simulink model "sim_model_simpledclink_2parallel_rlload"  (R2016a)
settings: Solver=ode4  StartTime=0.0  StopTime=Tfinal  FixedStep=Ts  RelTol=1e-3
values from neighbouring files (symbols this model uses):
  Cdc = 3*Cdc1    (= 1.5e-05)    [sim_parameters.m]    (also in sim_parameters_parallel.m; sim_parameters_rl_load.m)
  delta = acos(Ef/Vt)    [sim_parameters.m]    (also in sim_parameters_parallel.m; sim_parameters_rl_load.m = 0)
  deltad = delta*180/pi    [sim_parameters.m]    (also in sim_parameters_parallel.m; sim_parameters_rl_load.m = 0)
  ESL = 19e-9    (= 1.9e-08)    [sim_parameters.m]    (also in sim_parameters_parallel.m = 1.9e-14; sim_parameters_rl_load.m = 1e-15)
  ESR = 21.1e-15    (= 2.11e-14)    [sim_parameters_parallel.m]    (also in sim_parameters_rl_load.m = 1e-15)
  Lin = 1e-15    [sim_parameters_parallel.m]    (also in sim_parameters_rl_load.m = 1e-06)
  Lload = Xload/(2*pi*fout)    [sim_parameters_rl_load.m]
  ma = Vt*sqrt(3)/(Vdcm*0.612)    [sim_parameters.m]    (also in sim_parameters_parallel.m; sim_parameters_rl_load.m = 0.9)
  maxlim = 340    [sim_parameters.m]    (also in sim_parameters_parallel.m; sim_parameters_rl_load.m)
  minlim = 200    [sim_parameters.m]    (also in sim_parameters_parallel.m; sim_parameters_rl_load.m)
  phase = [0 90 0 90]    [sim_parameters.m]    (also in sim_parameters_parallel.m = [0 0]; sim_parameters_rl_load.m = [0 0])
  Rin = 1    [sim_parameters.m]    (also in sim_parameters_parallel.m = 50; sim_parameters_rl_load.m = 200)
  Ripth = 0.25    [sim_parameters.m]    (also in sim_parameters_parallel.m = 0.3; sim_parameters_rl_load.m = 0.03)
  Rload = Zload*pf    [sim_parameters_rl_load.m]
  Ts = 1e-6    (= 1e-06)    [sim_parameters.m]    (also in sim_parameters_parallel.m = 1e-07; sim_parameters_rl_load.m = 1e-08)
  Vin = Vdc + Rin*(Pout/Vdc)    (= 1751.48148148)    [sim_parameters_rl_load.m]
  wout = 2*pi*fout    (= 314.159265359)    [sim_parameters.m]    (also in sim_parameters_parallel.m; sim_parameters_rl_load.m)
libraries: powerlib x39, powerlib_meascontrol x26, simulink x2
settings Model: SimulationMode=accelerator  Creator=ugurm  LastModifiedBy=mesutto
settings DataIOCC: LimitDataPoints=on  SaveFormat=Array
settings DebuggingCC: UnderspecifiedInitializationDetection=Classic  MergeDetectMultiDrivingBlocksExec=none  SolverPrmCheckMsg=warning  StateNameClashWarn=warning
settings HardwareCC: ProdBitPerPointer=32  ProdLargestAtomicFloat=None  ProdIntDivRoundTo=Undefined  ProdEndianess=Unspecified  ProdWordSize=32  ProdHWDeviceType=32-bit Generic
settings ModelReferenceCC: PropagateSignalLabelsOutOfModel=off
settings ConfigComp: CovModelRefEnable=Off

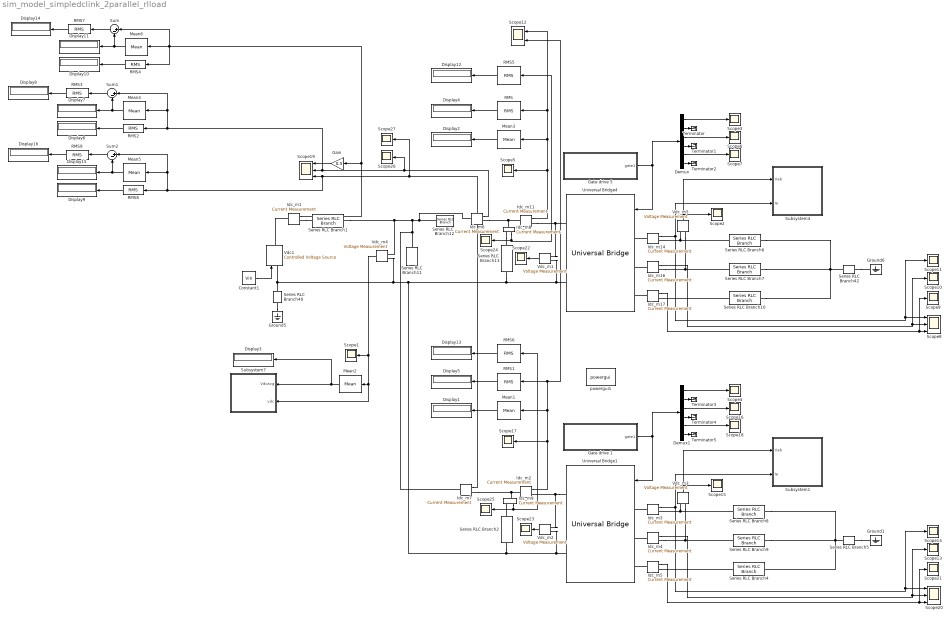
== system sim_model_simpledclink_2parallel_rlload ==
  Constant1 : Constant  Value=Vin
  Demux : Demux  Outputs=6
  Demux1 : Demux  Outputs=6
  Display{1..16} (16 alike) : Display
  Gain : Gain  Gain=0.5
  Gate drive 1 : Subsystem
  Gate drive 5 : Subsystem
  Ground1 : powerlib/Elements/Ground  LConnTagsString=a
  Ground5 : powerlib/Elements/Ground  LConnTagsString=a
  Ground6 : powerlib/Elements/Ground  LConnTagsString=a
  Idc_m{1..9,11,14,16..17} (13 alike) : powerlib/Measurements/Current Measurement  PhasorSimulation=off  OutputType=Complex  PSBequivalent=0
  Mean{1..6} (6 alike) : powerlib_meascontrol/Measurements/Mean  Freq=fout  Vinit=0  Ts=0
  RMS{,1..9} (10 alike) : powerlib_meascontrol/Measurements/RMS  TrueRMS=on  Freq=fout  RMSInit=0  Ts=0
  Scope{1..7,9..11,13..18,21..27} (23 alike) : Scope
  Scope12 : Scope  NumInputPorts=2
  Scope19 : Scope  NumInputPorts=3
  Scope20 : Scope  NumInputPorts=3
  Scope8 : Scope  NumInputPorts=3
  Series RLC Branch1 : powerlib/Elements/Series RLC Branch  LConnTagsString=__new0  RConnTagsString=__new0  BranchType=R  Resistance=Rin  Inductance=Lin  SetiL0=off  InitialCurrent=0  Capacitance=1e-6  Setx0=off  InitialVoltage=0  Measurements=None
  Series RLC Branch{4,6..10} (6 alike) : powerlib/Elements/Series RLC Branch  LConnTagsString=__new0  RConnTagsString=__new0  BranchType=RL  Resistance=Rload  Inductance=Lload  SetiL0=off  InitialCurrent=0  Capacitance=1e-6  Setx0=off  InitialVoltage=0  Measurements=None
  Series RLC Branch11 : powerlib/Elements/Series RLC Branch  LConnTagsString=__new0  RConnTagsString=__new0  BranchType=RL  Resistance=1e-3  Inductance=1e-6  SetiL0=off  InitialCurrent=0  Capacitance=1e-6  Setx0=off  InitialVoltage=0  Measurements=None
  Series RLC Branch12 : powerlib/Elements/Series RLC Branch  LConnTagsString=__new0  RConnTagsString=__new0  BranchType=RL  Resistance=1e-3  Inductance=1e-6  SetiL0=off  InitialCurrent=0  Capacitance=1e-6  Setx0=off  InitialVoltage=0  Measurements=None
  Series RLC Branch13 : powerlib/Elements/Series RLC Branch  LConnTagsString=__new0  RConnTagsString=__new0  BranchType=RLC  Resistance=ESR  Inductance=ESL  SetiL0=off  InitialCurrent=0  Capacitance=Cdc  Setx0=off  InitialVoltage=0  Measurements=None
  Series RLC Branch2 : powerlib/Elements/Series RLC Branch  LConnTagsString=__new0  RConnTagsString=__new0  BranchType=RLC  Resistance=ESR  Inductance=ESL  SetiL0=off  InitialCurrent=0  Capacitance=Cdc  Setx0=off  InitialVoltage=0  Measurements=None
  Series RLC Branch40 : powerlib/Elements/Series RLC Branch  LConnTagsString=__new0  RConnTagsString=__new0  BranchType=R  Resistance=1e12  Inductance=Lload  SetiL0=off  InitialCurrent=0  Capacitance=1e-6  Setx0=off  InitialVoltage=0  Measurements=None
  Series RLC Branch42 : powerlib/Elements/Series RLC Branch  LConnTagsString=__new0  RConnTagsString=__new0  BranchType=R  Resistance=1e12  Inductance=Lload  SetiL0=off  InitialCurrent=0  Capacitance=1e-6  Setx0=off  InitialVoltage=0  Measurements=None
  Series RLC Branch5 : powerlib/Elements/Series RLC Branch  LConnTagsString=__new0  RConnTagsString=__new0  BranchType=R  Resistance=1e12  Inductance=Lload  SetiL0=off  InitialCurrent=0  Capacitance=1e-6  Setx0=off  InitialVoltage=0  Measurements=None
  Subsystem1 : Subsystem
  Subsystem4 : Subsystem
  Subsystem7 : Subsystem
  Sum : Sum  Inputs=|+-
  Sum1 : Sum  Inputs=|+-
  Sum2 : Sum  Inputs=|+-
  Terminator{,1..5} (6 alike) : Terminator
  Universal Bridge1 : powerlib/Power Electronics/Universal Bridge  Arms=3  SnubberResistance=1e5  SnubberCapacitance=inf  Device=IGBT / Diodes  Ron=1e-6  Lon=0  ForwardVoltages="[  0  0  ]"  ForwardVoltage=0  GTOparameters=[ 10e-6 , 20e-6 ]  IGBTparameters=[0,0]  Measurements=None  Measurements_2=None  converterType=Rectifier
  Universal Bridge4 : powerlib/Power Electronics/Universal Bridge  Arms=3  SnubberResistance=1e5  SnubberCapacitance=inf  Device=IGBT / Diodes  Ron=1e-6  Lon=0  ForwardVoltages="[  0  0  ]"  ForwardVoltage=0  GTOparameters=[ 10e-6 , 20e-6 ]  IGBTparameters=[0,0]  Measurements=None  Measurements_2=None  converterType=Rectifier
  Vdc1 : powerlib/Electrical Sources/Controlled Voltage Source  Initialize=off  Source_Type=DC  Amplitude=200  Phase=0  Frequency=0  Measurements=None
  Vdc_m{1..5} (5 alike) : powerlib/Measurements/Voltage Measurement  PhasorSimulation=off  OutputType=Complex  PSBequivalent=0
  powergui1 : powerlib/powergui  Priority=1  SimulationMode=Discrete  SolverType=Tustin  SampleTime=Ts  frequency=60  SPID=off  DisableSnubberDevices=off  DisableRonSwitches=off  DisableVfSwitches=off  SwTol=0  DisplayEquations=off  Interpol=off  ExternalGateDelay=off  methode=off  Ts=0  FunctionMessages=off  echomessages=off  HookPort=off  EnableUseOfTLC=off  x0status=blocks  frequencyindice=0  Pbase=100e6  ErrMax=1e-4  Iterations=50  UnitsV=kV  UnitsW=MW  buscounter=0  RestoreLinks=warning  ResistiveCurrentMeasurement=off  Frange=[0:2:500]  Ylog=off  Xlog=on  ShowGrid=off  save=off  variable=ZData  structure=vdc  ZoomFFT=off  StartTime=0.35  cycles=5  DisplayStyle=4  fundamental=50  FreqAxis=off  MaxFrequency=50000  frequencyindicesteady=1  RmsSteady=1  display=off
  wires:
  Gate drive 5/1(gate1) -> Universal Bridge4/1, Demux/1
  Vdc_m5/1 -> Subsystem4/1(Vab), Scope2/1
  Idc_m14/1 -> Subsystem4/2(Ia), Scope11/1, Scope8/1
  Constant1/1 -> Vdc1/1
  Idc_m16/1 -> Scope10/1, Scope8/2
  Idc_m17/1 -> Scope9/1, Scope8/3
  Idc_m11/1 -> Mean3/1, RMS/1, Scope12/1, Scope5/1
  Mean3/1 -> Display2/1
  RMS/1 -> Display4/1
  Demux/1 -> Scope3/1
  Demux/5 -> Scope7/1
  Demux/3 -> Scope6/1
  Demux/2 -> Terminator/1
  Demux/4 -> Terminator1/1
  Demux/6 -> Terminator2/1
  Mean2/1 -> Display3/1, Subsystem7/1(Vdcavg)
  Gate drive 1/1(gate1) -> Universal Bridge1/1, Demux1/1
  Vdc_m3/1 -> Subsystem1/1(Vab), Scope15/1
  Idc_m3/1 -> Subsystem1/2(Ia), Scope14/1, Scope20/1
  Idc_m4/1 -> Scope13/1, Scope20/2
  Idc_m5/1 -> Scope21/1, Scope20/3
  Idc_m2/1 -> Mean1/1, Scope12/2, RMS1/1, Scope17/1
  Mean1/1 -> Display1/1
  RMS1/1 -> Display5/1
  Demux1/1 -> Scope4/1
  Demux1/5 -> Scope18/1
  Demux1/3 -> Scope16/1
  Demux1/2 -> Terminator3/1
  Demux1/4 -> Terminator4/1
  Demux1/6 -> Terminator5/1
  Vdc_m4/1 -> Scope1/1, Subsystem7/2(vdc), Mean2/1
  Gain/1 -> Scope19/1
  Vdc_m1/1 -> Scope22/1
  Vdc_m2/1 -> Scope23/1
  Idc_m8/1 -> RMS5/1, Scope24/1
  Idc_m6/1 -> Sum1/1, Mean4/1, RMS2/1, Scope19/2, Scope26/1
  RMS4/1 -> Display10/1
  Idc_m1/1 -> Sum/1, RMS4/1, Mean6/1, Gain/1
  Mean6/1 -> Display11/1, Sum/2
  RMS5/1 -> Display12/1
  RMS6/1 -> Display13/1
  Idc_m9/1 -> RMS6/1, Scope25/1
  Sum/1 -> RMS7/1
  RMS7/1 -> Display14/1
  RMS2/1 -> Display6/1
  Mean4/1 -> Display7/1, Sum1/2
  Sum1/1 -> RMS3/1
  RMS3/1 -> Display8/1
  RMS8/1 -> Display9/1
  Idc_m7/1 -> Scope27/1, Mean5/1, Sum2/1, RMS8/1, Scope19/3
  Mean5/1 -> Display15/1, Sum2/2
  Sum2/1 -> RMS9/1
  RMS9/1 -> Display16/1
  connections:
  Vdc_m5/LConn1 -- Series RLC Branch6/LConn1 -- Idc_m14/RConn1
  Series RLC Branch42/RConn1 -- Ground6/LConn1
  Series RLC Branch40/RConn1 -- Ground5/LConn1
  Idc_m14/LConn1 -- Universal Bridge4/LConn1
  Series RLC Branch42/LConn1 -- Series RLC Branch7/RConn1 -- Series RLC Branch10/RConn1 -- Series RLC Branch6/RConn1
  Idc_m16/LConn1 -- Universal Bridge4/LConn2
  Idc_m17/LConn1 -- Universal Bridge4/LConn3
  Series RLC Branch10/LConn1 -- Idc_m17/RConn1
  Idc_m16/RConn1 -- Series RLC Branch7/LConn1 -- Vdc_m5/LConn2
  Idc_m11/RConn1 -- Vdc_m1/LConn1 -- Universal Bridge4/RConn1
  Idc_m1/RConn1 -- Series RLC Branch1/LConn1
  Idc_m1/LConn1 -- Vdc1/RConn1
  Idc_m3/RConn1 -- Series RLC Branch8/LConn1 -- Vdc_m3/LConn1
  Vdc_m3/LConn2 -- Series RLC Branch9/LConn1 -- Idc_m4/RConn1
  Universal Bridge4/RConn2 -- Vdc_m1/LConn2 -- Series RLC Branch13/RConn1 -- Series RLC Branch2/RConn1 -- Universal Bridge1/RConn2 -- Vdc_m2/LConn2 -- Vdc_m4/LConn2 -- Vdc1/LConn1 -- Series RLC Branch40/LConn1
  Universal Bridge1/RConn1 -- Idc_m2/RConn1 -- Vdc_m2/LConn1
  Idc_m7/RConn1 -- Idc_m9/LConn1 -- Idc_m2/LConn1
  Idc_m3/LConn1 -- Universal Bridge1/LConn1
  Idc_m4/LConn1 -- Universal Bridge1/LConn2
  Series RLC Branch4/LConn1 -- Idc_m5/RConn1
  Idc_m5/LConn1 -- Universal Bridge1/LConn3
  Series RLC Branch5/RConn1 -- Ground1/LConn1
  Idc_m6/RConn1 -- Idc_m8/LConn1 -- Idc_m11/LConn1
  Vdc_m4/LConn1 -- Series RLC Branch1/RConn1 -- Idc_m6/LConn1 -- Series RLC Branch12/LConn1 -- Idc_m7/LConn1 -- Series RLC Branch11/RConn1
  Series RLC Branch8/RConn1 -- Series RLC Branch9/RConn1 -- Series RLC Branch5/LConn1 -- Series RLC Branch4/RConn1
  Idc_m8/RConn1 -- Series RLC Branch13/LConn1
  Series RLC Branch2/LConn1 -- Idc_m9/RConn1

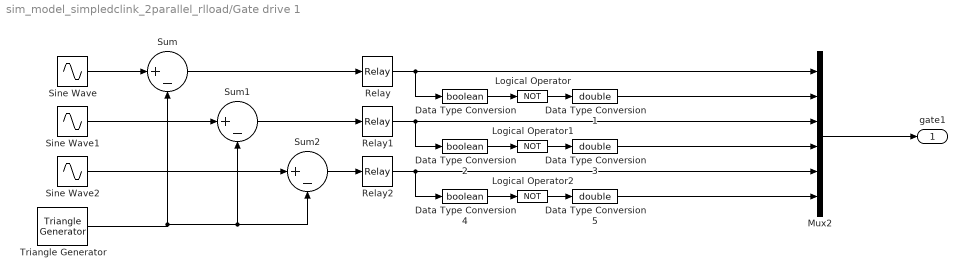
== system sim_model_simpledclink_2parallel_rlload/Gate drive 1 ==
  Data Type Conversion : DataTypeConversion  OutDataTypeStr=boolean
  Data Type Conversion1 : DataTypeConversion  OutDataTypeStr=double
  Data Type Conversion2 : DataTypeConversion  OutDataTypeStr=boolean
  Data Type Conversion3 : DataTypeConversion  OutDataTypeStr=double
  Data Type Conversion4 : DataTypeConversion  OutDataTypeStr=boolean
  Data Type Conversion5 : DataTypeConversion  OutDataTypeStr=double
  Logical Operator : Logic  Operator=NOT  AllPortsSameDT=off  OutDataTypeStr=boolean
  Logical Operator1 : Logic  Operator=NOT  AllPortsSameDT=off  OutDataTypeStr=boolean
  Logical Operator2 : Logic  Operator=NOT  AllPortsSameDT=off  OutDataTypeStr=boolean
  Mux2 : Mux  Inputs=6
  Relay : Relay
  Relay1 : Relay
  Relay2 : Relay
  Sine Wave : Sin  Amplitude=ma  Frequency=wout  Phase=delta  SampleTime=0
  Sine Wave1 : Sin  Amplitude=ma  Frequency=wout  Phase=-2*pi/3+delta  SampleTime=0
  Sine Wave2 : Sin  Amplitude=ma  Frequency=wout  Phase=2*pi/3+delta  SampleTime=0
  Sum : Sum  Inputs=|+-
  Sum1 : Sum  Inputs=|+-
  Sum2 : Sum  Inputs=|+-
  Triangle Generator : powerlib_meascontrol/Pulse & Signal Generators/Triangle Generator  Freq=fsw  Phase=phase(2)  Ts=Ts
  gate1 : Outport
  wires:
  Sine Wave/1 -> Sum/1
  Triangle Generator/1 -> Sum1/2, Sum2/2, Sum/2
  Sine Wave1/1 -> Sum1/1
  Sine Wave2/1 -> Sum2/1
  Sum/1 -> Relay/1
  Sum1/1 -> Relay1/1
  Sum2/1 -> Relay2/1
  Data Type Conversion/1 -> Logical Operator/1
  Relay/1 -> Data Type Conversion/1, Mux2/1
  Logical Operator/1 -> Data Type Conversion1/1
  Data Type Conversion1/1 -> Mux2/2
  Data Type Conversion2/1 -> Logical Operator1/1
  Relay1/1 -> Data Type Conversion2/1, Mux2/3
  Logical Operator1/1 -> Data Type Conversion3/1
  Data Type Conversion3/1 -> Mux2/4
  Data Type Conversion4/1 -> Logical Operator2/1
  Relay2/1 -> Data Type Conversion4/1, Mux2/5
  Logical Operator2/1 -> Data Type Conversion5/1
  Data Type Conversion5/1 -> Mux2/6
  Mux2/1 -> gate1/1

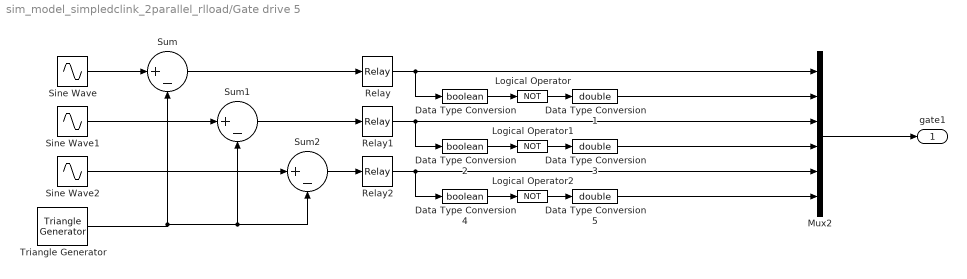
== system sim_model_simpledclink_2parallel_rlload/Gate drive 5 ==
  Data Type Conversion : DataTypeConversion  OutDataTypeStr=boolean
  Data Type Conversion1 : DataTypeConversion  OutDataTypeStr=double
  Data Type Conversion2 : DataTypeConversion  OutDataTypeStr=boolean
  Data Type Conversion3 : DataTypeConversion  OutDataTypeStr=double
  Data Type Conversion4 : DataTypeConversion  OutDataTypeStr=boolean
  Data Type Conversion5 : DataTypeConversion  OutDataTypeStr=double
  Logical Operator : Logic  Operator=NOT  AllPortsSameDT=off  OutDataTypeStr=boolean
  Logical Operator1 : Logic  Operator=NOT  AllPortsSameDT=off  OutDataTypeStr=boolean
  Logical Operator2 : Logic  Operator=NOT  AllPortsSameDT=off  OutDataTypeStr=boolean
  Mux2 : Mux  Inputs=6
  Relay : Relay
  Relay1 : Relay
  Relay2 : Relay
  Sine Wave : Sin  Amplitude=ma  Frequency=wout  Phase=delta  SampleTime=0
  Sine Wave1 : Sin  Amplitude=ma  Frequency=wout  Phase=-2*pi/3+delta  SampleTime=0
  Sine Wave2 : Sin  Amplitude=ma  Frequency=wout  Phase=2*pi/3+delta  SampleTime=0
  Sum : Sum  Inputs=|+-
  Sum1 : Sum  Inputs=|+-
  Sum2 : Sum  Inputs=|+-
  Triangle Generator : powerlib_meascontrol/Pulse & Signal Generators/Triangle Generator  Freq=fsw  Phase=phase(1)  Ts=Ts
  gate1 : Outport
  wires:
  Sine Wave/1 -> Sum/1
  Triangle Generator/1 -> Sum1/2, Sum2/2, Sum/2
  Sine Wave1/1 -> Sum1/1
  Sine Wave2/1 -> Sum2/1
  Sum/1 -> Relay/1
  Sum1/1 -> Relay1/1
  Sum2/1 -> Relay2/1
  Data Type Conversion/1 -> Logical Operator/1
  Relay/1 -> Data Type Conversion/1, Mux2/1
  Logical Operator/1 -> Data Type Conversion1/1
  Data Type Conversion1/1 -> Mux2/2
  Data Type Conversion2/1 -> Logical Operator1/1
  Relay1/1 -> Data Type Conversion2/1, Mux2/3
  Logical Operator1/1 -> Data Type Conversion3/1
  Data Type Conversion3/1 -> Mux2/4
  Data Type Conversion4/1 -> Logical Operator2/1
  Relay2/1 -> Data Type Conversion4/1, Mux2/5
  Logical Operator2/1 -> Data Type Conversion5/1
  Data Type Conversion5/1 -> Mux2/6
  Mux2/1 -> gate1/1

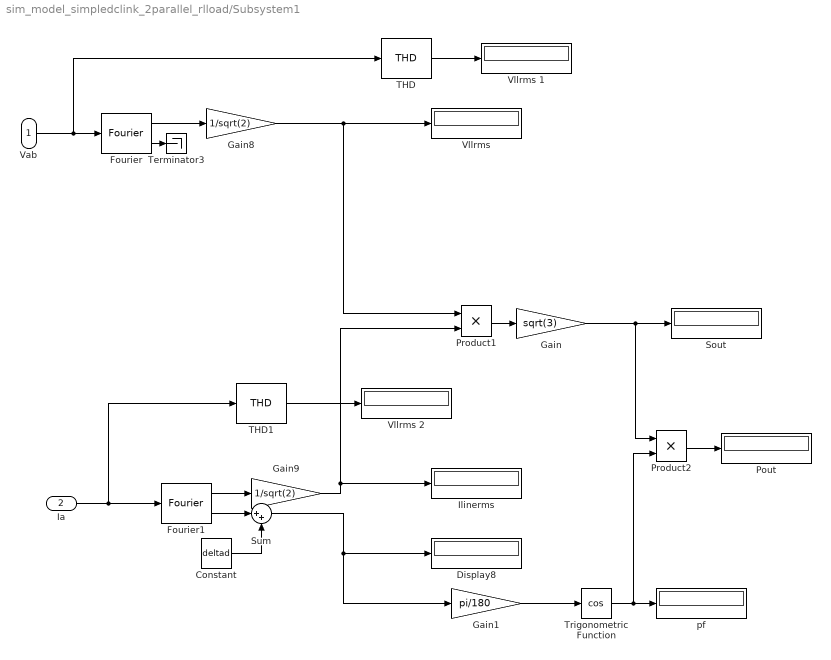
== system sim_model_simpledclink_2parallel_rlload/Subsystem1 ==
  Vab : Inport
  Ia : Inport  Port=2
  Constant : Constant  Value=deltad
  Display8 : Display
  Fourier : powerlib_meascontrol/Measurements/Fourier  Freq=fout  n=1  InInit=[0, 0]  Ts=Ts
  Fourier1 : powerlib_meascontrol/Measurements/Fourier  Freq=fout  n=1  InInit=[0, 0]  Ts=Ts
  Gain : Gain  Gain=sqrt(3)
  Gain1 : Gain  Gain=pi/180
  Gain8 : Gain  Gain=1/sqrt(2)
  Gain9 : Gain  Gain=1/sqrt(2)
  "Ilinerms " : Display
  Pout : Display
  Product1 : Product
  Product2 : Product
  Sout : Display
      settings: Format=short_e
  Sum : Sum  Inputs=|++
  THD : powerlib_meascontrol/Measurements/THD  Freq=fout  Ts=0
  THD1 : powerlib_meascontrol/Measurements/THD  Freq=fout  Ts=0
  Terminator3 : Terminator
  Trigonometric Function : Trigonometry  Operator=cos
  "Vllrms " : Display
  Vllrms 1 : Display
  Vllrms 2 : Display
  pf : Display
  wires:
  Gain8/1 -> Product1/1, "Vllrms "/1
  Gain9/1 -> "Ilinerms "/1, Product1/2
  Ia/1 -> THD1/1, Fourier1/1
  Fourier1/1 -> Gain9/1
  Vab/1 -> THD/1, Fourier/1
  Fourier/1 -> Gain8/1
  Product1/1 -> Gain/1
  Gain/1 -> Product2/1, Sout/1
  Sum/1 -> Gain1/1, Display8/1
  Trigonometric Function/1 -> Product2/2, pf/1
  Gain1/1 -> Trigonometric Function/1
  Product2/1 -> Pout/1
  Fourier/2 -> Terminator3/1
  THD/1 -> Vllrms 1/1
  THD1/1 -> Vllrms 2/1
  Fourier1/2 -> Sum/1
  Constant/1 -> Sum/2

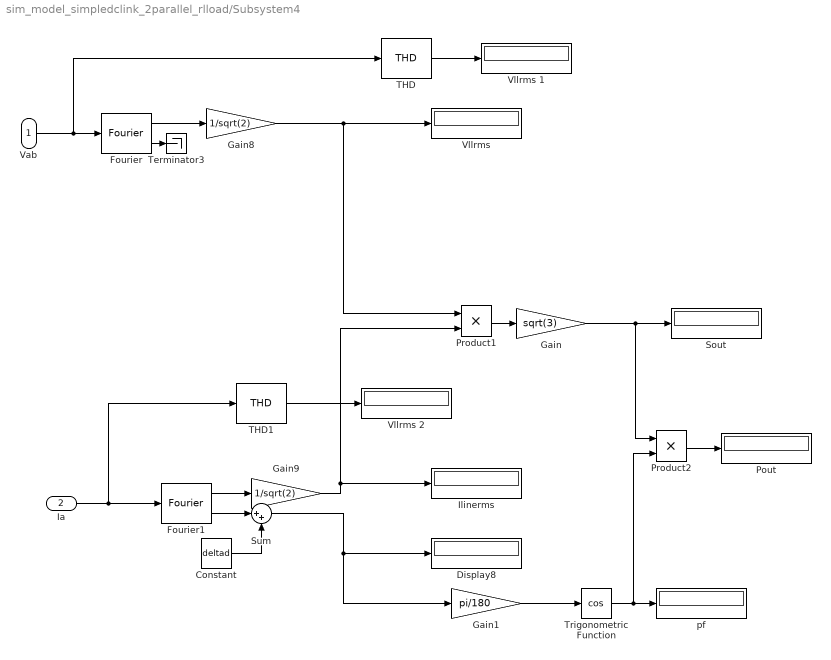
== system sim_model_simpledclink_2parallel_rlload/Subsystem4 ==
  Vab : Inport
  Ia : Inport  Port=2
  Constant : Constant  Value=deltad
  Display8 : Display
  Fourier : powerlib_meascontrol/Measurements/Fourier  Freq=fout  n=1  InInit=[0, 0]  Ts=Ts
  Fourier1 : powerlib_meascontrol/Measurements/Fourier  Freq=fout  n=1  InInit=[0, 0]  Ts=Ts
  Gain : Gain  Gain=sqrt(3)
  Gain1 : Gain  Gain=pi/180
  Gain8 : Gain  Gain=1/sqrt(2)
  Gain9 : Gain  Gain=1/sqrt(2)
  "Ilinerms " : Display
  Pout : Display
  Product1 : Product
  Product2 : Product
  Sout : Display
      settings: Format=short_e
  Sum : Sum  Inputs=|++
  THD : powerlib_meascontrol/Measurements/THD  Freq=fout  Ts=0
  THD1 : powerlib_meascontrol/Measurements/THD  Freq=fout  Ts=0
  Terminator3 : Terminator
  Trigonometric Function : Trigonometry  Operator=cos
  "Vllrms " : Display
  Vllrms 1 : Display
  Vllrms 2 : Display
  pf : Display
  wires:
  Gain8/1 -> Product1/1, "Vllrms "/1
  Gain9/1 -> "Ilinerms "/1, Product1/2
  Ia/1 -> THD1/1, Fourier1/1
  Fourier1/1 -> Gain9/1
  Vab/1 -> THD/1, Fourier/1
  Fourier/1 -> Gain8/1
  Product1/1 -> Gain/1
  Gain/1 -> Product2/1, Sout/1
  Sum/1 -> Gain1/1, Display8/1
  Trigonometric Function/1 -> Product2/2, pf/1
  Gain1/1 -> Trigonometric Function/1
  Product2/1 -> Pout/1
  Fourier/2 -> Terminator3/1
  THD/1 -> Vllrms 1/1
  THD1/1 -> Vllrms 2/1
  Fourier1/2 -> Sum/1
  Constant/1 -> Sum/2

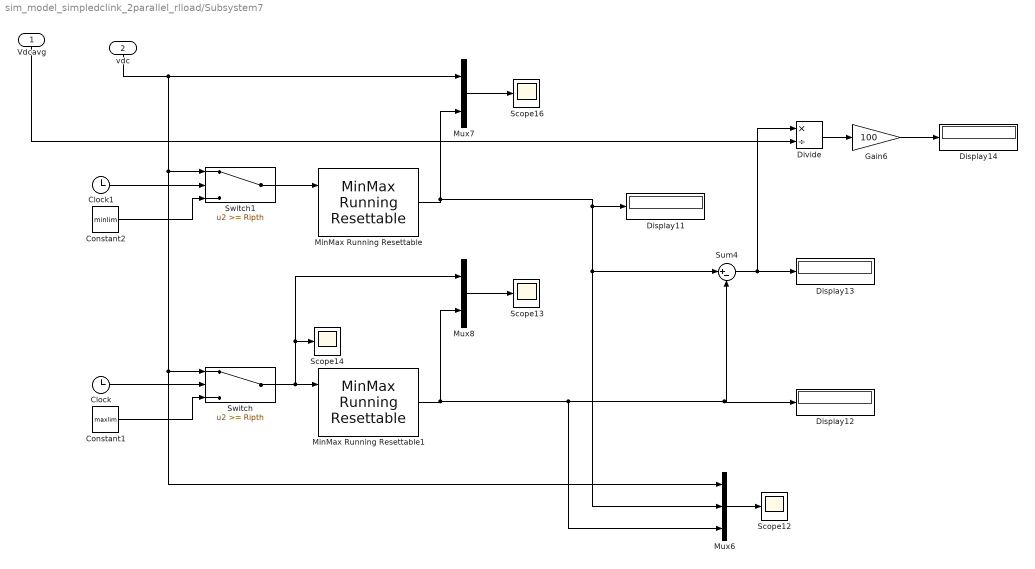
== system sim_model_simpledclink_2parallel_rlload/Subsystem7 ==
  Vdcavg : Inport
  vdc : Inport  Port=2
  Clock : Clock
  Clock1 : Clock
  Constant1 : Constant  Value=maxlim  SampleTime=Ts
  Constant2 : Constant  Value=minlim  SampleTime=Ts
  Display{11..14} (4 alike) : Display
  Divide : Product  Inputs=*/
  Gain6 : Gain  Gain=100
  MinMax Running Resettable : simulink/Math Operations/MinMax Running Resettable  Function=max  vinit=0.0
  MinMax Running Resettable1 : simulink/Math Operations/MinMax Running Resettable  Function=min  vinit=700
  Mux6 : Mux  Inputs=3
  Mux7 : Mux  Inputs=2
  Mux8 : Mux  Inputs=2
  Scope{12..14,16} (4 alike) : Scope
  Sum4 : Sum  Inputs=|+-
  Switch : Switch  Threshold=Ripth
  Switch1 : Switch  Threshold=Ripth
  wires:
  MinMax Running Resettable/1 -> Display11/1, Mux6/2, Sum4/1, Mux7/2
  Clock/1 -> Switch/2
  Mux8/1 -> Scope13/1
  Gain6/1 -> Display14/1
  Constant1/1 -> Switch/3
  MinMax Running Resettable1/1 -> Mux6/3, Display12/1, Sum4/2, Mux8/2
  Mux7/1 -> Scope16/1
  Switch/1 -> Mux8/1, Scope14/1, MinMax Running Resettable1/1
  Sum4/1 -> Divide/1, Display13/1
  Divide/1 -> Gain6/1
  Mux6/1 -> Scope12/1
  Vdcavg/1 -> Divide/2
  vdc/1 -> Mux7/1, Switch1/1, Mux6/1, Switch/1
  Switch1/1 -> MinMax Running Resettable/1
  Clock1/1 -> Switch1/2
  Constant2/1 -> Switch1/3
